simulink model "PROGRAM_COUNTER_02"  (R2022a)
settings: Solver=VariableStepAuto  StartTime=0.0  StopTime=10.0  RelTol=1e-3
undefined symbols (not defined in the file or in its folder): xc7z010iclg225
libraries: hdlBasic x1933, hlsBasic x1, vmcUtilities x1
(part 1 of 12)
settings Model: Creator=sebas  LastModifiedBy=sebas

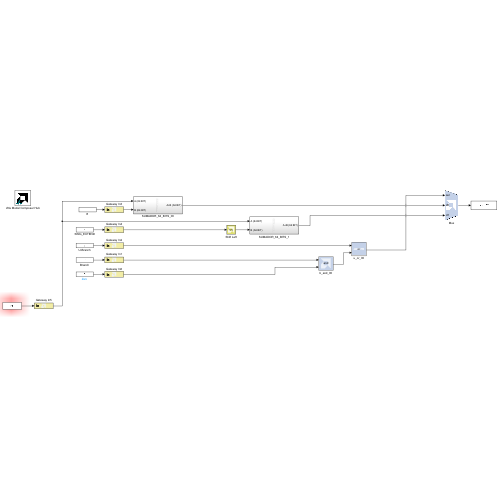
[thumbnail: Simulink's stored preview of the top-level diagram]
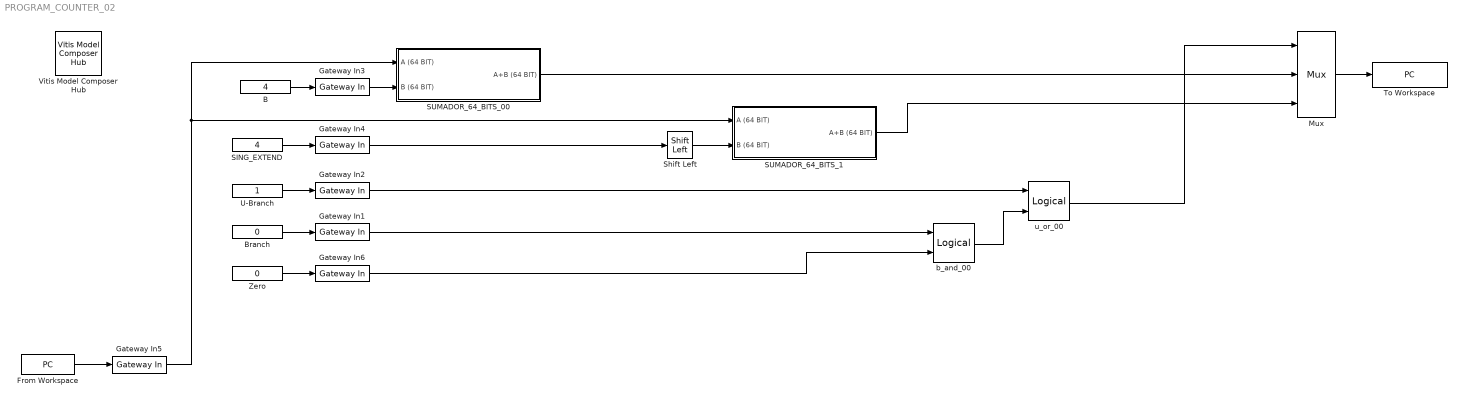
== system PROGRAM_COUNTER_02 ==
  B : Constant  Value=4
  Branch : Constant  Value=0
  From Workspace : FromWorkspace  VariableName=PC
  Gateway In{1..6} (6 alike) : hdlBasic/Gateway In  gui_display_data_type=Fixed-point  arith_type=Unsigned  n_bits=1  bin_pt=0  preci_type=Single  exp_width=8  frac_width=24  rows=1  columns=1  quantization="Round  (unbiased: +/- Inf)"  overflow=Saturate  period=1  UseAsADC=off  ADCChannel='1'  interface=None  automatic_assignment=on  address_offset=hex2dec('00')  intf_name=''  intf_description=''  default_value=0  timing_constraint=None  locs_specified=off  LOCs={}  io_standard={}  inherit_from_input=off  hdl_port=on  XmcBlockStatus=1  maskContainerNames=group4  block_type=gatewayin  block_config=sysgen:gateway_in_config  block_width_w=590  block_height_w=620  block_width=640  block_height=850
  Mux : hdlBasic/Mux  inputs=2  en=off  latency=0  precision=Full  arith_type=Unsigned  n_bits=16  bin_pt=14  quantization=Truncate  overflow=Wrap  XmcBlockStatus=1  maskContainerNames=tabcontainer1  block_type=mux  block_config=sysgen:Mux_config
  SING_EXTEND : Constant  Value=4
  SUMADOR_64_BITS_00 : Subsystem
  SUMADOR_64_BITS_1 : Subsystem
  Shift Left : hlsBasic/Shift Left  ShiftAmount=2
  To Workspace : ToWorkspace  VariableName=PC  SaveFormat=Timeseries  SampleTime=-1
  U-Branch : Constant
  Vitis Model Composer Hub : vmcUtilities/Vitis Model Composer Hub  Tag=genX  CodeGeneration=off  TargetDirectory=./code  ExportType=AI Engines  IpVendor=xilinx.com  IpLibrary=hls  IpVersion=1.0  IpHWLanguage=Verilog  AieCompilerOptions={}  AieSimulatorOptions={}  CreateTestbench=off  TestbenchStackSize=10  RunAieSim=off  AieSimTimeout=50000  RunAieSimProfiling=off  LaunchVitisAnalyzer=off  PlotOutput=off  RunX86Sim=off  X86SimTimeout=10  GenHwImage=off  PlatformType=Not Specified  HwSystemType=Baremetal  HwValidationTarget=hw  ProjDevice=xc7z010iclg225-1L  ProjDevicePart=xc7z010iclg225-1L  SamplePeriod=-1  ClockFrequency=200  DataPathParallelism=1  xilinxfamily=zynq  part=xc7z010i  speed=-1L  package=clg225  directory=./netlist  testbench=off  incr_netlist=off  synthesis_tool=Vivado  clock_wrapper=Clock Enables  dbl_ovrd=According to Block Masks  dcm_input_clock_period=10  sysclk_period=10  simulink_period=1  eval_field=0  LogFileName=''  NThreads=4
  Zero : Constant  Value=0
  b_and_00 : hdlBasic/Logical  logical_function=AND  inputs=2  en=off  latency=0  precision=Full  arith_type=Unsigned  n_bits=16  bin_pt=0  align_bp=on  overflow=[]  quantization=[]  XmcBlockStatus=1  maskContainerNames=tabcontainer1  block_type=logical  block_config=sysgen:Logical_config
  u_or_00 : hdlBasic/Logical  logical_function=OR  inputs=2  en=off  latency=0  precision=Full  arith_type=Unsigned  n_bits=16  bin_pt=0  align_bp=on  overflow=[]  quantization=[]  XmcBlockStatus=1  maskContainerNames=tabcontainer1  block_type=logical  block_config=sysgen:Logical_config
  wires:
  Branch/1 -> Gateway In1/1
  Gateway In5/1 -> SUMADOR_64_BITS_1/1(A (64 BIT)), SUMADOR_64_BITS_00/1(A (64 BIT))
  SUMADOR_64_BITS_00/1(A+B (64 BIT)) -> Mux/2
  SUMADOR_64_BITS_1/1(A+B (64 BIT)) -> Mux/3
  U-Branch/1 -> Gateway In2/1
  b_and_00/1 -> u_or_00/2
  Gateway In2/1 -> u_or_00/1
  Gateway In1/1 -> b_and_00/1
  u_or_00/1 -> Mux/1
  Shift Left/1 -> SUMADOR_64_BITS_1/2(B (64 BIT))
  B/1 -> Gateway In3/1
  Gateway In3/1 -> SUMADOR_64_BITS_00/2(B (64 BIT))
  Gateway In4/1 -> Shift Left/1
  SING_EXTEND/1 -> Gateway In4/1
  From Workspace/1 -> Gateway In5/1
  Mux/1 -> To Workspace/1
  Zero/1 -> Gateway In6/1
  Gateway In6/1 -> b_and_00/2
